simulink model "SWS_1b"  (R2023a)
settings: Solver=ode4  StartTime=0.0  StopTime=30  FixedStep=0.005  RelTol=1e-3
InitFcn:
  | SWS
values from neighbouring files (symbols this model uses):
  K_scheduled = zeros(length(V_op), 2)    [CAL3.m]    (also in CUB.m; DLC2.m; MUS.m; OHZ.m)
  V_op = 5:5:85    [CAL3.m]    (also in CUB.m; DLC2.m; MUS.m; OHZ.m)
  X_track = [linspace(0, runway_length, 200)'; runway_length + R_track * cos(theta_circ(2:end))]    [CAL3.m]    (also in CUB.m = [0; 5000]; DLC2.m = 0:0.1:total_track_length; MUS.m = [0; 2000]; OHZ.m = [0; 2000])
  Y_track = [zeros(200, 1); R_track + R_track * sin(theta_circ(2:end))]    [CAL3.m]    (also in CUB.m = [0; 0]; DLC2.m = zeros(size(X_track)); MUS.m = [0; 0]; OHZ.m = [0; 0])
libraries: simulink x2, slpidlib x2
(part 3 of 3)

== matlab function SWS_1b/Vehicle & Powertrain Plant1/MATLAB Function ==
  data: delta input; Trr_m input; Trl_m input; Trr_f input; Trl_f input; Tf_f input; vx input; vy input; r input; psi input; SOC input; T_batt input; T_motor input; w_fl input; w_fr input; w_rl input; w_rr input; vx_dot output; vy_dot output; r_dot output; X_dot output; Y_dot output; psi_dot output; s_dot output; SOC_dot output; T_batt_dot output; T_mot_dot output; Fz_f_tot output; Fz_r_tot output; Fz_rl output; Fz_rr output; Fx_vec output; Fy_vec output; Fz_vec output; w_vec output; w_dot_vec output; veh_params parameter
function [vx_dot, vy_dot, r_dot, X_dot, Y_dot, psi_dot, s_dot, SOC_dot, T_batt_dot, T_mot_dot, Fz_f_tot, Fz_r_tot, Fz_rl, Fz_rr, Fx_vec, Fy_vec, Fz_vec, w_vec, w_dot_vec] = vehicle_physics_engine(delta, Trr_m, Trl_m, Trr_f, Trl_f, Tf_f, vx, vy, r, psi, SOC, T_batt, T_motor, w_fl, w_fr, w_rl, w_rr, veh_params)
    % =========================================================================
    % STABLE BASELINE 7-DOF PLANAR PHYSICS (Zero Roll/Pitch Delay)
    % =========================================================================
    
    % 1. UNPACK PARAMETERS
    m = veh_params.m; Iz = veh_params.Iz; lf = veh_params.lf; lr = veh_params.lr; L = veh_params.L;
    tw = veh_params.tw; h_cg = veh_params.h_cg; Rw = veh_params.Rw; Iw = veh_params.Iw; 
    G = veh_params.G; g = veh_params.g; rho = veh_params.rho; CdA = veh_params.CdA;
    roll_bias_f = veh_params.roll_bias_f; mu_max = veh_params.mu_max; C_rr = veh_params.C_rr;
    ks_f = veh_params.ks_f; ks_r = veh_params.ks_r; C_tire = veh_params.C_tire; E_tire = veh_params.E_tire;
    
    if abs(vx) < 0.5, vx_safe = 0.5 * sign(vx + 1e-6); else, vx_safe = vx; end
    F_aero_drag = 0.5 * rho * CdA * vx_safe * abs(vx_safe);

    % ---------------------------------------------------------------------
    % 2. INSTANTANEOUS WEIGHT TRANSFER (QUASI-STATIC)
    % ---------------------------------------------------------------------
    Fx_total_tq = (Trr_m + Trl_m)*G + Trr_f + Trl_f + Tf_f;
    ax_inst = (Fx_total_tq/Rw - F_aero_drag) / m;
    ay_inst = vx_safe * r;
    
    dFz_x = m * ax_inst * (h_cg / L);
    dFz_y = m * ay_inst * (h_cg / tw);
    
    Fz_f_tot = m * g * (lr / L) - dFz_x;
    Fz_r_tot = m * g * (lf / L) + dFz_x;
    
    % Instant distribution based on static roll bias
    Fz_fl = max(100, Fz_f_tot/2 - dFz_y * roll_bias_f);
    Fz_fr = max(100, Fz_f_tot/2 + dFz_y * roll_bias_f);
    Fz_rl = max(100, Fz_r_tot/2 - dFz_y * (1 - roll_bias_f));
    Fz_rr = max(100, Fz_r_tot/2 + dFz_y * (1 - roll_bias_f));
    Fz_vec = [Fz_fl, Fz_fr, Fz_rl, Fz_rr];
    
    % ---------------------------------------------------------------------
    % 3. PACEJKA COMBINED SLIP
    % ---------------------------------------------------------------------
    B_f = ks_f / (C_tire * mu_max * (Fz_f_tot/2 + 1e-6)); 
    B_r = ks_r / (C_tire * mu_max * (Fz_r_tot/2 + 1e-6)); 
    
    v_hub_fl = vx_safe - (tw / 2) * r; v_hub_fr = vx_safe + (tw / 2) * r;
    v_hub_rl = vx_safe - (tw / 2) * r; v_hub_rr = vx_safe + (tw / 2) * r;
    
    k_fl = (w_fl * Rw - v_hub_fl) / max(abs(v_hub_fl), 1.0);
    k_fr = (w_fr * Rw - v_hub_fr) / max(abs(v_hub_fr), 1.0);
    k_rl = (w_rl * Rw - v_hub_rl) / max(abs(v_hub_rl), 1.0);
    k_rr = (w_rr * Rw - v_hub_rr) / max(abs(v_hub_rr), 1.0);
    
    alpha_fl = delta - atan((vy + lf * r) / max(abs(v_hub_fl), 1.0));
    alpha_fr = delta - atan((vy + lf * r) / max(abs(v_hub_fr), 1.0));
    alpha_rl = -atan((vy - lr * r) / max(abs(v_hub_rl), 1.0));
    alpha_rr = -atan((vy - lr * r) / max(abs(v_hub_rr), 1.0));
    
    sigma_fl = sqrt(k_fl^2 + tan(alpha_fl)^2) + 1e-6;
    sigma_fr = sqrt(k_fr^2 + tan(alpha_fr)^2) + 1e-6;
    sigma_rl = sqrt(k_rl^2 + tan(alpha_rl)^2) + 1e-6;
    sigma_rr = sqrt(k_rr^2 + tan(alpha_rr)^2) + 1e-6;
    
    F_tot_fl = mu_max * Fz_fl * sin(C_tire * atan(B_f * sigma_fl - E_tire * (B_f * sigma_fl - atan(B_f * sigma_fl))));
    F_tot_fr = mu_max * Fz_fr * sin(C_tire * atan(B_f * sigma_fr - E_tire * (B_f * sigma_fr - atan(B_f * sigma_fr))));
    F_tot_rl = mu_max * Fz_rl * sin(C_tire * atan(B_r * sigma_rl - E_tire * (B_r * sigma_rl - atan(B_r * sigma_rl))));
    F_tot_rr = mu_max * Fz_rr * sin(C_tire * atan(B_r * sigma_rr - E_tire * (B_r * sigma_rr - atan(B_r * sigma_rr))));
    
    Fx_fl = F_tot_fl * (k_fl / sigma_fl) - C_rr * Fz_fl * tanh(v_hub_fl * 10);
    Fx_fr = F_tot_fr * (k_fr / sigma_fr) - C_rr * Fz_fr * tanh(v_hub_fr * 10);
    Fx_rl = F_tot_rl * (k_rl / sigma_rl) - C_rr * Fz_rl * tanh(v_hub_rl * 10);
    Fx_rr = F_tot_rr * (k_rr / sigma_rr) - C_rr * Fz_rr * tanh(v_hub_rr * 10);
    Fx_vec = [Fx_fl, Fx_fr, Fx_rl, Fx_rr];
    
    Fy_fl = F_tot_fl * (tan(alpha_fl) / sigma_fl);
    Fy_fr = F_tot_fr * (tan(alpha_fr) / sigma_fr);
    Fy_rl = F_tot_rl * (tan(alpha_rl) / sigma_rl);
    Fy_rr = F_tot_rr * (tan(alpha_rr) / sigma_rr);
    Fy_vec = [Fy_fl, Fy_fr, Fy_rl, Fy_rr];
    
    % 4. CHASSIS INTEGRATORS
    w_fl_dot = (-abs(Tf_f/2)*sign(w_fl) - Fx_fl*Rw)/Iw;
    w_fr_dot = (-abs(Tf_f/2)*sign(w_fr) - Fx_fr*Rw)/Iw;
    w_rl_dot = (Trl_m*G - abs(Trl_f)*sign(w_rl) - Fx_rl*Rw)/Iw;
    w_rr_dot = (Trr_m*G - abs(Trr_f)*sign(w_rr) - Fx_rr*Rw)/Iw;
    w_dot_vec = [w_fl_dot, w_fr_dot, w_rl_dot, w_rr_dot];
    w_vec = [w_fl, w_fr, w_rl, w_rr];
    
    sum_Fx = (Fx_fl + Fx_fr)*cos(delta) - (Fy_fl + Fy_fr)*sin(delta) + Fx_rl + Fx_rr;
    vx_dot = (sum_Fx - F_aero_drag)/m + vy*r;
    sum_Fy = (Fy_fl + Fy_fr)*cos(delta) + (Fx_fl + Fx_fr)*sin(delta) + Fy_rl + Fy_rr;
    vy_dot = sum_Fy/m - vx_safe*r;
    
    r_dot = (lf*((Fy_fl + Fy_fr)*cos(delta) + (Fx_fl + Fx_fr)*sin(delta)) - lr*(Fy_rl + Fy_rr) + (Fx_rr - Fx_rl)*(tw/2))/Iz;
    
    X_dot = vx_safe*cos(psi) - vy*sin(psi);
    Y_dot = vx_safe*sin(psi) + vy*cos(psi);
    psi_dot = r; s_dot = vx_safe;
    
    % THERMALS & SOC (Simplified Baseline)
    P_mech = (Trr_m + Trl_m)*G*(vx_safe/Rw);
    I_curr = (P_mech / 0.90) / veh_params.V_pack;
    SOC_dot = -I_curr/(veh_params.Cap_Ah*3600);
    T_batt_dot = ((I_curr^2)*veh_params.R_pack - veh_params.hA_cool_batt*(T_batt-veh_params.T_coolant_batt))/(veh_params.m_batt*veh_params.cp_batt);
    T_mot_dot  = (abs(P_mech*0.1) - veh_params.hA_cool_motor*(T_motor-veh_params.T_ambient))/(veh_params.m_motor*veh_params.cp_motor);
end
